simulink model "LQGrocket"  (R2020a)
settings: Solver=FixedStepAuto  StartTime=0.0  StopTime=120  FixedStep=Ts  RelTol=1e-3  EnableMultiTasking=on
values from neighbouring files (symbols this model uses):
  Ad = sysd.a    [rocket_main_LQG.m]
  Bd = sysd.b(:,1:3)    [rocket_main_LQG.m]
  Bwd = sysd.b(:,4)    [rocket_main_LQG.m]
  Cd = sysd.c    [rocket_main_LQG.m]
  inic = [10 0 1000 0 deg2rad(-10) 0]'    [rocket_main_LQG.m]
  Rv = (0.3^2)*eye(3)    [rocket_main_LQG.m]
  Rw = 0.1^2    (= 0.01)    [rocket_main_LQG.m]
  Ts = .001    (= 0.001)    [rocket_main_LQG.m]
undefined symbols (not defined in the file or in its folder): Kdlqr, Kss
libraries: simulink_extras x1
settings Model: Creator=nagamune  LastModifiedBy=jchia
settings DataIOCC: LimitDataPoints=on  SaveFormat=Array  ReturnWorkspaceOutputs=off
settings OptimizationCC: LifeSpan=inf
settings DebuggingCC: SolverPrmCheckMsg=warning  SFUnexpectedBacktrackingDiag=warning  SFNoUnconditionalDefaultTransitionDiag=warning  SFExecutionAtInitializationDiag=none  ArithmeticOperatorsInVariantConditions=warning
settings HardwareCC: ProdBitPerPointer=32  ProdBitPerSizeT=32  ProdBitPerPtrDiffT=32  ProdLargestAtomicFloat=None  ProdIntDivRoundTo=Undefined  ProdEndianess=Unspecified  ProdWordSize=32  ProdHWDeviceType=32-bit Generic
settings ModelReferenceCC: PropagateSignalLabelsOutOfModel=off
settings SFSimCC: SimUseLocalCustomCode=off  CustomCodeUndefinedFunction=UseInterfaceOnly
settings RTWCC: RTWUseLocalCustomCode=off
settings CodeAppCC: StateflowObjectComments=on
settings GRTTargetCC: TargetLangStandard=C89/C90 (ANSI)
settings ConfigComp: CovMetricSettings=dw  CovSaveCumulativeToWorkspaceVar=on  CovSaveSingleToWorkspaceVar=on  CovExternalEMLEnable=off  CovSFcnEnable=off

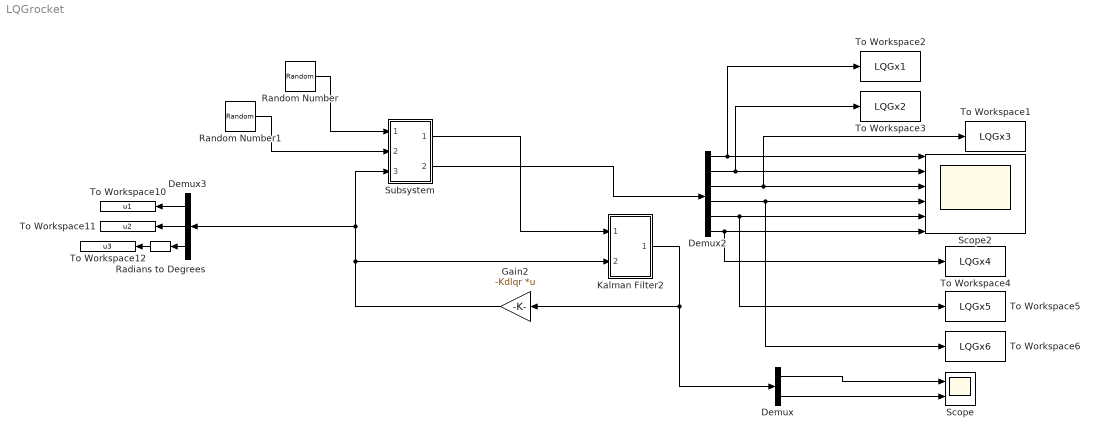
== system LQGrocket ==
  Demux : Demux  Outputs=2
  Demux2 : Demux  Outputs=6
  Demux3 : Demux  Outputs=3
  Gain2 : Gain  Gain=-Kdlqr  Multiplication=Matrix(K*u)  SampleTime=Ts
  Kalman Filter2 : Subsystem
  Radians to Degrees : simulink_extras/Transformations/Radians to Degrees
  Random Number : RandomNumber  Variance=Rw  SampleTime=Ts
  Random Number1 : RandomNumber  Variance=Rv  SampleTime=Ts
  Scope : Scope  NumInputPorts=2
  Scope2 : Scope  NumInputPorts=6
  Subsystem : Subsystem
  To Workspace1 : ToWorkspace  VariableName=LQGx3  SaveFormat=Timeseries  SampleTime=-1
  To Workspace10 : ToWorkspace  VariableName=u1  SaveFormat=Timeseries  SampleTime=-1
  To Workspace11 : ToWorkspace  VariableName=u2  SaveFormat=Timeseries  SampleTime=-1
  To Workspace12 : ToWorkspace  VariableName=u3  SaveFormat=Timeseries  SampleTime=-1
  To Workspace2 : ToWorkspace  VariableName=LQGx1  SaveFormat=Timeseries  SampleTime=-1
  To Workspace3 : ToWorkspace  VariableName=LQGx2  SaveFormat=Timeseries  SampleTime=-1
  To Workspace4 : ToWorkspace  VariableName=LQGx4  SaveFormat=Timeseries  SampleTime=-1
  To Workspace5 : ToWorkspace  VariableName=LQGx5  SaveFormat=Timeseries  SampleTime=-1
  To Workspace6 : ToWorkspace  VariableName=LQGx6  SaveFormat=Timeseries  SampleTime=-1
  wires:
  Demux2/2 -> Scope2/2, To Workspace3/1
  Demux2/1 -> To Workspace2/1, Scope2/1
  Subsystem/1(Out1) -> Kalman Filter2/1(In1)
  Random Number1/1 -> Subsystem/2(In2)
  Subsystem/2(Out2) -> Demux2/1
  Demux/2 -> Scope/2
  Kalman Filter2/1(Out1) -> Demux/1, Gain2/1
  Demux/1 -> Scope/1
  Random Number/1 -> Subsystem/1(In1)
  Demux2/3 -> To Workspace1/1, Scope2/3
  Demux2/4 -> To Workspace6/1, Scope2/4
  Demux2/5 -> To Workspace5/1, Scope2/5
  Demux2/6 -> To Workspace4/1, Scope2/6
  Demux3/1 -> To Workspace10/1
  Demux3/3 -> Radians to Degrees/1
  Gain2/1 -> Subsystem/3(In3), Demux3/1, Kalman Filter2/2(In2)
  Radians to Degrees/1 -> To Workspace12/1
  Demux3/2 -> To Workspace11/1

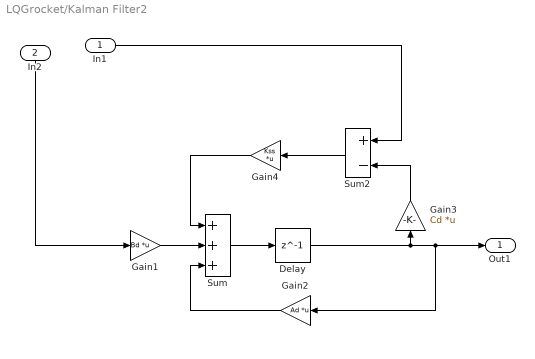
== system LQGrocket/Kalman Filter2 ==
  In1 : Inport
  In2 : Inport  Port=2
  Delay : Delay  DelayLength=1  InitialCondition=inic  SampleTime=Ts
  Gain1 : Gain  Gain=Bd  Multiplication=Matrix(K*u)  SampleTime=Ts
  Gain2 : Gain  Gain=Ad  Multiplication=Matrix(K*u)  SampleTime=Ts
  Gain3 : Gain  Gain=Cd  Multiplication=Matrix(K*u)  SampleTime=Ts
  Gain4 : Gain  Gain=Kss  Multiplication=Matrix(K*u)  SampleTime=Ts
  Sum : Sum  Inputs=+++  SampleTime=Ts
  Sum2 : Sum  Inputs=+-  SampleTime=Ts
  Out1 : Outport
  wires:
  Gain2/1 -> Sum/3
  Delay/1 -> Out1/1, Gain2/1, Gain3/1
  Sum/1 -> Delay/1
  Gain1/1 -> Sum/2
  Gain3/1 -> Sum2/2
  Sum2/1 -> Gain4/1
  In1/1 -> Sum2/1
  In2/1 -> Gain1/1
  Gain4/1 -> Sum/1

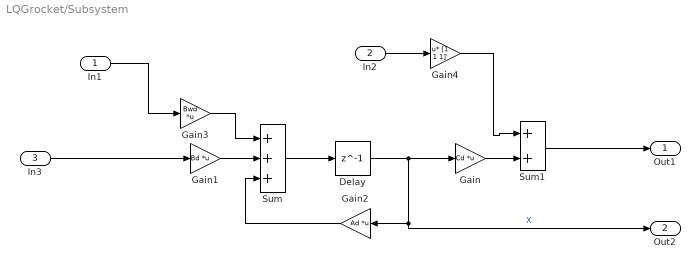
== system LQGrocket/Subsystem ==
  In1 : Inport
  In2 : Inport  Port=2
  In3 : Inport  Port=3
  Delay : Delay  DelayLength=1  InitialCondition=inic  SampleTime=Ts
  Gain : Gain  Gain=Cd  Multiplication=Matrix(K*u)  SampleTime=Ts
  Gain1 : Gain  Gain=Bd  Multiplication=Matrix(K*u)  SampleTime=Ts
  Gain2 : Gain  Gain=Ad  Multiplication=Matrix(K*u)  SampleTime=Ts
  Gain3 : Gain  Gain=Bwd  Multiplication=Matrix(K*u)  SampleTime=Ts
  Gain4 : Gain  Gain=[1 1 1]'  Multiplication=Matrix(u*K)  SampleTime=Ts
  Sum : Sum  Inputs=+++  SampleTime=Ts
  Sum1 : Sum  SampleTime=Ts
  Out1 : Outport
  Out2 : Outport  Port=2
  wires:
  Gain3/1 -> Sum/1
  Delay/1 -> Out2/1, Gain2/1, Gain/1  "X"
  Sum/1 -> Delay/1
  Gain2/1 -> Sum/3
  Gain/1 -> Sum1/2
  In3/1 -> Gain1/1
  Gain1/1 -> Sum/2
  In1/1 -> Gain3/1
  Sum1/1 -> Out1/1
  In2/1 -> Gain4/1
  Gain4/1 -> Sum1/1
